simulink model "project_2_part2_ex1"  (R2026a)
settings: Solver=FixedStepAuto  StopTime=Tfin  FixedStep=1e-3  MaxStep=1e-2  MinStep=1e-3  RelTol=5e-3
values from neighbouring files (symbols this model uses):
  ze0 = [X0;Y0;psi0;vx0;vy0;wpsi0]    [part2.m]
settings Model: PacingRate=0.750000  Creator=The MathWorks, Inc.  LastModifiedBy=matte
settings SolverCC: ZeroCrossAlgorithm=Adaptive  DecoupledContinuousIntegration=on  MinimalZcImpactIntegration=on
settings DataIOCC: SaveFormat=StructureWithTime
settings OptimizationCC: BufferReuse=off
settings ConfigComp: PLC_TargetIDE=codesys35  PLC_MultiTBSigbuilderTimeRange=off  PLC_FoldFBCallOutputVar=off  PLC_RemoveUnusedSSMethodCallArguments=off  PLC_UseCallOutputArgSyntax=off  PLC_EnableUnsignedAndDoubleTypes=off  PLC_EnableUDTSplitting=off  PLC_MaxFieldsInUDT=500.0  PLC_InlineEnumCastFunction=off  PLC_RTWMaxIdLength=31.0  PLC_RollThreshold=5.0  PLC_ActiveTab=0.0  PLC_EnableStringLiteralTB=on  PLC_Enable64bitIntSupport=off

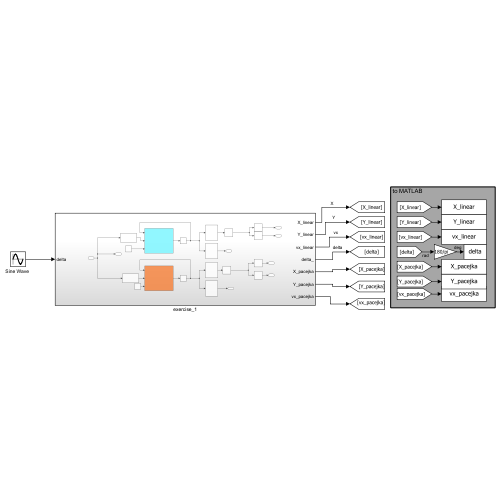
[thumbnail: Simulink's stored preview of the top-level diagram]
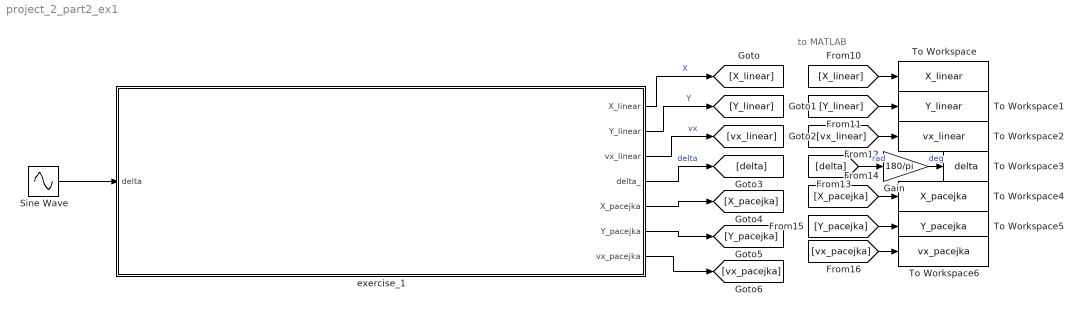
== system project_2_part2_ex1 ==
  note: to MATLAB
  Gain : Gain  Gain=180/pi
  "Sine Wave " : Sin  Amplitude=0.5  Frequency=0.2  SampleTime=0
  To Workspace : ToWorkspace  VariableName=X_linear  SaveFormat=Timeseries  SampleTime=-1
  To Workspace1 : ToWorkspace  VariableName=Y_linear  SaveFormat=Timeseries  SampleTime=-1
  To Workspace2 : ToWorkspace  VariableName=vx_linear  SaveFormat=Timeseries  SampleTime=-1
  To Workspace3 : ToWorkspace  VariableName=delta  SaveFormat=Timeseries  SampleTime=-1
  To Workspace4 : ToWorkspace  VariableName=X_pacejka  SaveFormat=Timeseries  SampleTime=-1
  To Workspace5 : ToWorkspace  VariableName=Y_pacejka  SaveFormat=Timeseries  SampleTime=-1
  To Workspace6 : ToWorkspace  VariableName=vx_pacejka  SaveFormat=Timeseries  SampleTime=-1
  exercise_1 : Subsystem
  wires:
  exercise_1/1(X_linear) -> [X_linear]  "X"
  exercise_1/2(Y_linear) -> [Y_linear]  "Y"
  exercise_1/3(vx_linear) -> [vx_linear]  "vx"
  exercise_1/4(delta_) -> [delta]  "delta"
  "Sine Wave "/1 -> exercise_1/1(delta)
  exercise_1/5(X_pacejka) -> [X_pacejka]
  exercise_1/6(Y_pacejka) -> [Y_pacejka]
  exercise_1/7(vx_pacejka) -> [vx_pacejka]
  [X_linear] -> To Workspace/1
  [Y_linear] -> To Workspace1/1
  [vx_linear] -> To Workspace2/1
  [X_pacejka] -> To Workspace4/1
  [Y_pacejka] -> To Workspace5/1
  [vx_pacejka] -> To Workspace6/1
  [delta] -> Gain/1  "rad"
  Gain/1 -> To Workspace3/1  "deg"

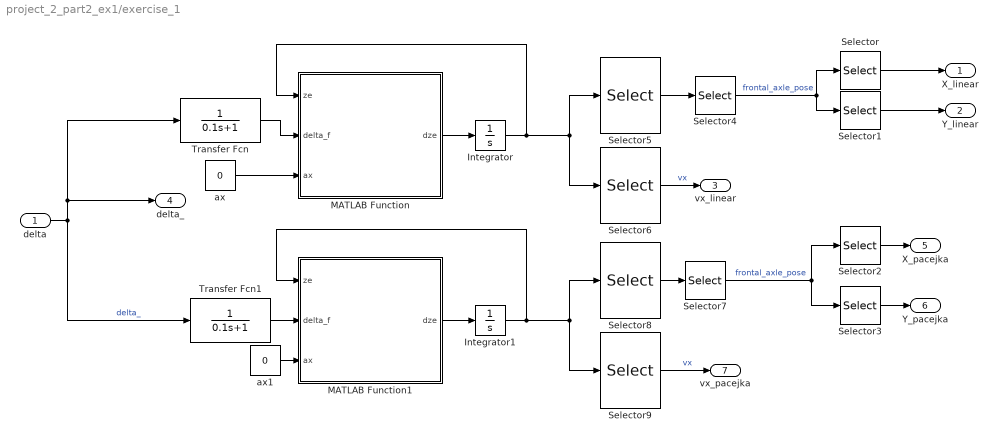
== system project_2_part2_ex1/exercise_1 ==
  delta : Inport
  Integrator : Integrator  InitialCondition=ze0
  Integrator1 : Integrator  InitialCondition=ze0
  MATLAB Function : MATLAB Function  TreatAsAtomicUnit=on
  MATLAB Function1 : MATLAB Function  TreatAsAtomicUnit=on
  Selector : Selector  InputPortWidth=2  IndexOptions=Index vector (dialog)  Indices=1  OutputSizes=1
  Selector1 : Selector  InputPortWidth=2  IndexOptions=Index vector (dialog)  Indices=2  OutputSizes=1
  Selector2 : Selector  InputPortWidth=2  IndexOptions=Index vector (dialog)  Indices=1  OutputSizes=1
  Selector3 : Selector  InputPortWidth=2  IndexOptions=Index vector (dialog)  Indices=2  OutputSizes=1
  Selector4 : Selector  InputPortWidth=3  IndexOptions=Index vector (dialog)  Indices=[1 2]  OutputSizes=1
  Selector5 : Selector  InputPortWidth=6  IndexOptions=Index vector (dialog)  Indices=[1:3]  OutputSizes=1
  Selector6 : Selector  InputPortWidth=6  IndexOptions=Index vector (dialog)  Indices=4  OutputSizes=1
  Selector7 : Selector  InputPortWidth=3  IndexOptions=Index vector (dialog)  Indices=[1 2]  OutputSizes=1
  Selector8 : Selector  InputPortWidth=6  IndexOptions=Index vector (dialog)  Indices=[1:3]  OutputSizes=1
  Selector9 : Selector  InputPortWidth=6  IndexOptions=Index vector (dialog)  Indices=4  OutputSizes=1
  Transfer Fcn : TransferFcn  Denominator=[0.1 1]
  Transfer Fcn1 : TransferFcn  Denominator=[0.1 1]
  ax : Constant  Value=0
  ax1 : Constant  Value=0
  X_linear : Outport
  Y_linear : Outport  Port=2
  vx_linear : Outport  Port=3
  delta_ : Outport  Port=4
  X_pacejka : Outport  Port=5
  Y_pacejka : Outport  Port=6
  vx_pacejka : Outport  Port=7
  wires:
  Selector1/1 -> Y_linear/1
  Selector/1 -> X_linear/1
  Selector4/1 -> Selector1/1, Selector/1  "frontal_axle_pose"
  Selector6/1 -> vx_linear/1  "vx"
  Selector9/1 -> vx_pacejka/1  "vx"
  Selector7/1 -> Selector3/1, Selector2/1  "frontal_axle_pose"
  Selector2/1 -> X_pacejka/1
  Selector3/1 -> Y_pacejka/1
  delta/1 -> Transfer Fcn1/1, Transfer Fcn/1, delta_/1  "delta_"
  MATLAB Function/1(dze) -> Integrator/1
  Transfer Fcn/1 -> MATLAB Function/2(delta_f)
  Selector5/1 -> Selector4/1
  ax/1 -> MATLAB Function/3(ax)
  Integrator/1 -> Selector6/1, Selector5/1, MATLAB Function/1(ze)
  MATLAB Function1/1(dze) -> Integrator1/1
  Selector8/1 -> Selector7/1
  Transfer Fcn1/1 -> MATLAB Function1/2(delta_f)
  ax1/1 -> MATLAB Function1/3(ax)
  Integrator1/1 -> MATLAB Function1/1(ze), Selector8/1, Selector9/1

== matlab function project_2_part2_ex1/exercise_1/MATLAB Function1 ==
  data: ze input; delta_f input; dze output; ax input
function dze = DSTP_nonlinear_model(ze,delta_f, ax)

% States
X = ze(1);
Y =ze(2);
psi = ze(3);
vx = ze(4);
vy = ze(5);
wpsi = ze(6);

% % Inputs
% ax    = u(1);
% delta_f = u(2);

% Vehicle parameters:
l1 = 1.2;       % m
l2 = 1.6;       % m
m = 1575;       % kg
Jz = 4000;      % kg*m^2
C1 = 27e3;      % N/rad
C2 = C1;

% Slip angles (non-linear model)
alpha1 = atan((vy + l1*wpsi)/vx) - delta_f;
alpha2 = atan((vy - l2*wpsi)/vx);

% Pacejka's tire model
[fp_alpha1, fp_alpha2] = pacejka_model(alpha1,alpha2,C1,C2);
Fy1 = -fp_alpha1 * cos(delta_f);
Fy2 = -fp_alpha2;

% State equations
dX    = vx*cos(psi) - vy*sin(psi);
dY    = vx*sin(psi) + vy*cos(psi);
dpsi  = wpsi;
dvx   = vy*wpsi + ax;
dvy   = -vx*wpsi + (2/m)*(Fy1 + Fy2);
dwpsi = (2/Jz)*(l1*Fy1 - l2*Fy2);

dze = [dX; dY; dpsi; dvx; dvy; dwpsi];

% Pacejka Lateral tire forces 
function [fp_alpha1, fp_alpha2] = pacejka_model(alpha1,alpha2,C1,C2)

% Tire parameters:
p1 = 3863;      % N
p2 = 1.5;
p4 = -0.5;
p3_front = C1/p1/p2;  % front tire
p3_rear = C2/p1/p2;   % rear tire

fp_alpha1 = p1*sin(p2*atan(p3_front*alpha1 - p4*(p3_front*alpha1 - atan(p3_front*alpha1))));
fp_alpha2 = p1*sin(p2*atan(p3_rear*alpha2 - p4*(p3_rear*alpha2 - atan(p3_rear*alpha2))));

end
end

== matlab function project_2_part2_ex1/exercise_1/MATLAB Function ==
  data: ze input; delta_f input; dze output; ax input
function dze = DST_linear_model(ze,delta_f, ax)

% States
X = ze(1);
Y =ze(2);
psi = ze(3);
vx = ze(4);
vy = ze(5);
wpsi = ze(6);

% % Inputs
% ax    = u(1);
% delta_f = u(2);

% Vehicle parameters:
l1 = 1.2;       % m
l2 = 1.6;       % m
m = 1575;       % kg
Jz = 4000;      % kg*m^2
C1 = 27e3;      % N/rad
C2 = C1;        % N/rad

% Slip angles (linear model)
alpha1 = (vy + l1*wpsi)/vx - delta_f;
alpha2 = (vy - l2*wpsi)/vx;

% Lateral tire forces
Fy1 = -C1 * alpha1;
Fy2 = -C2 * alpha2;

% Equations of motion
dX    = vx*cos(psi) - vy*sin(psi);
dY    = vx*sin(psi) + vy*cos(psi);
dpsi  = wpsi;
dvx   = vy*wpsi + ax;
dvy   = -vx*wpsi + (2/m)*(Fy1 + Fy2);
dwpsi = (2/Jz)*(l1*Fy1 - l2*Fy2);

dze = [dX; dY; dpsi; dvx; dvy; dwpsi];
end
